simulink model "Wheel_Speed"  (R2020b)
settings: Solver=VariableStepAuto  StartTime=0.0  StopTime=25  RelTol=1e-3
undefined symbols (not defined in the file): I, Kf, PBmax, Rr, TB, v0
settings Model: Creator=Shantam Garg  LastModifiedBy=Shantam Garg
settings DataIOCC: SaveOutput=off  SaveTime=off

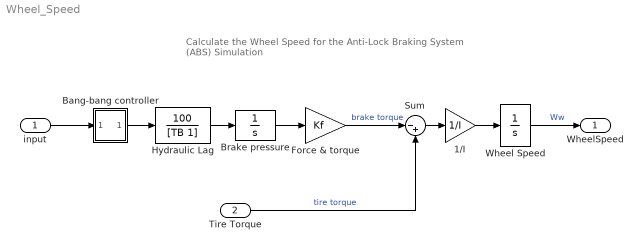
== system Wheel_Speed ==
  note: Calculate the Wheel Speed for the
      | Anti-Lock Braking System (ABS) Simulation
  input : Inport  OutDataTypeStr=double  PortDimensions=1  SampleTime=0
  Tire Torque : Inport  Port=2  OutDataTypeStr=double  PortDimensions=1  SampleTime=0
  1/I : Gain  Gain=1/I  SaturateOnIntegerOverflow=on  OutDataTypeStr=Inherit: Same as input  ParamDataTypeStr=Inherit: Same as input
  Bang-bang controller : Subsystem  mask(Sign){}
      mask help: y = sign(x)
      mask Help: Sign Function:\n\t\t\ty = 1 if x > 0\n\t\t\ty = 0 if x = 0\n\t\t\ty = -1 if x < 0
      mask Display: plot(-50,-50,50,50,[-50,50],[0,0],[0,0],[-50,50],[-40,0],[-30,-30],[0,40],[30,30])
  Brake pressure : Integrator  LimitOutput=on  UpperSaturationLimit=PBmax  LowerSaturationLimit=0
  Force & torque : Gain  Gain=Kf  SaturateOnIntegerOverflow=on  OutDataTypeStr=Inherit: Same as input  ParamDataTypeStr=Inherit: Same as input
  "Hydraulic Lag " : TransferFcn  Numerator=[100]  Denominator=[TB 1]
  Sum : Sum  Inputs=|-+  InputSameDT=on  SaturateOnIntegerOverflow=on  OutDataTypeStr=Inherit: Same as first input
  Wheel Speed : Integrator  InitialCondition=v0/Rr  LimitOutput=on  UpperSaturationLimit=1000  LowerSaturationLimit=0
  WheelSpeed : Outport  OutDataTypeStr=double  PortDimensions=1  SampleTime=0  VectorParamsAs1DForOutWhenUnconnected=off
  wires:
  1/I/1 -> Wheel Speed/1
  Force & torque/1 -> Sum/1  "brake torque"
  Bang-bang controller/1(out_1) -> "Hydraulic Lag "/1
  Tire Torque/1 -> Sum/2  "tire torque"
  Sum/1 -> 1/I/1
  input/1 -> Bang-bang controller/1(in_1)
  Brake pressure/1 -> Force & torque/1
  Wheel Speed/1 -> WheelSpeed/1  "Ww"
  "Hydraulic Lag "/1 -> Brake pressure/1

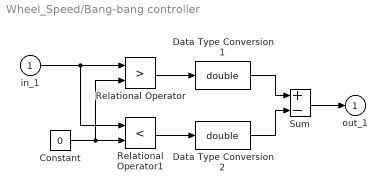
== system Wheel_Speed/Bang-bang controller ==
  in_1 : Inport
  Constant : Constant  Value=0
  Data Type Conversion1 : DataTypeConversion  OutDataTypeStr=double  SaturateOnIntegerOverflow=on  RndMeth=Zero
  Data Type Conversion2 : DataTypeConversion  OutDataTypeStr=double  SaturateOnIntegerOverflow=on  RndMeth=Zero
  Relational Operator : RelationalOperator  Operator=>  OutDataTypeStr=boolean  RndMeth=Nearest  InputSameDT=on
  Relational Operator1 : RelationalOperator  Operator=<  OutDataTypeStr=boolean  RndMeth=Nearest  InputSameDT=on
  Sum : Sum  Inputs=+-  InputSameDT=on  SaturateOnIntegerOverflow=on  OutDataTypeStr=Inherit: Same as first input
  out_1 : Outport  InitialOutput=0  VectorParamsAs1DForOutWhenUnconnected=off
  wires:
  Data Type Conversion2/1 -> Sum/2
  Data Type Conversion1/1 -> Sum/1
  Sum/1 -> out_1/1
  Relational Operator/1 -> Data Type Conversion1/1
  Relational Operator1/1 -> Data Type Conversion2/1
  Constant/1 -> Relational Operator/2, Relational Operator1/2
  in_1/1 -> Relational Operator1/1, Relational Operator/1
